simulink model "Track_model_wtihtesting_datacooling"  (R2024a)
settings: Solver=FixedStepAuto  StartTime=0.0  StopTime=1200  FixedStep=0.01  MaxStep=1e-2  MinStep=1e-5  RelTol=1e-3  AbsTol=1e-11
PreLoadFcn:
  | Straight1_Track = [75	3.446	29.063	1.834	47.653	8.247	3.373	13.154	57.193	39.54	5.916	3.204	2.701	2.747	90.673	4.72	3.366	94.658	23.788	1	40.161	15.969	17.891	3.717	36.358	76.419	54.208	36.993	4.775	55.007	1.783	4.349
  | ];
  | Curved_Track = [13.325	13.688	13.825	14.949	16.182	52.505	18.752	19.67	17.192	18.934	14.945	16.948	14.677	9.353	16.047	6.011	19.463	14.821	17.716	9.886	20.496	17.101	19.463	24.351	37.401	18.473	21.711	5.558	59.024	6.989	13.452	41.008
  | ];
  | Radius1 = [12	16.8	16.75	13.5	18.6	22.46	17.818	17.73	14	25.6	16.44	15.538	14.4	26.75	44.307	40	20.44	27.09	18.18	23.42	22.933	36.75	14.631	39	27.714	18.667	15.778	21.2	22.927	27.67	24.4	27.778
  | ];
model workspace (MAT data in the model file):
  Curve_Track = [19 13 16.3 21 23 16.5 21.6 28.81 24.6 43.9 54.836 13.8]
  Straight_Track = [35.7 53.5 32.527 50 30 20 11.2 36.6 21.4 41 38.7 74.5]
  Trac_vel = [10 5 8 12 8 9 10 9 11 14 10 10]
(part 1 of 2)
settings Model: Creator=91933  LastModifiedBy=Lenovo
settings SolverCC: MaxConsecutiveMinStep=10000000
settings DebuggingCC: UnconnectedInputMsg=warning  UnconnectedOutputMsg=warning  UnconnectedLineMsg=warning
settings ModelReferenceCC: EnableRefExpFcnMdlSchedulingChecks=on
settings RTWCC: GPUComputeCapability=3.5  DLArmComputeVersion=19.05

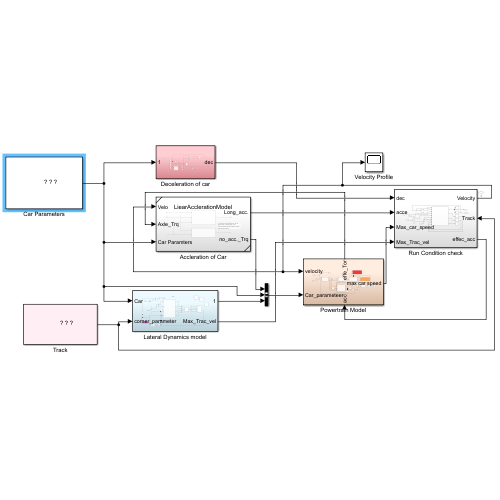
[thumbnail: Simulink's stored preview of the top-level diagram]
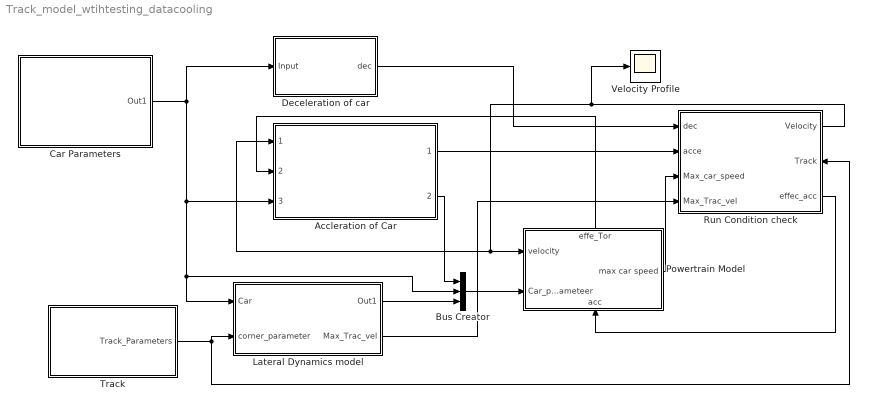
== system Track_model_wtihtesting_datacooling ==
  Accleration of Car : Subsystem  ReferencedSubsystem=LiearAcclerationModel
  Bus Creator : BusCreator  Inputs=3
  Car Parameters : Subsystem
      mask Display: image('C:\Users\91933\Pictures\IMG_5657.JPG'); % Use "Edit Image" on toolstrip to change.
  Deceleration of car : Subsystem
  Lateral Dynamics model : Subsystem
  Powertrain Model : Subsystem
      settings: PortSchema="{\"entries\":[{\"content\":{\"sides\":[{\"content\":{\"connectorIds\":[\"In1\",\"In2\"]},\"type\":\"ConnectorPlacement.EquallySpacedRectSide\",\"uuid\":\"7a6424a8-f57f-46b7-98ad-5f26a9320d27\"},{\"content\":{\"connectorIds\":[\"Out1\"],\"side\":\"RIGHT\"},\"type\":\"ConnectorPlacement.EquallySpacedRectSide\",\"uuid\":\"30370c1c-7325-4103-814a-5db3cbc3461c\"},{\"content\":{\"connectorIds\":[\"Out2\"],\"side\":\"TOP\"},\"type\":\"ConnectorPlacement.EquallySpacedRectSide\",\"uuid\":\"7e814e0a-36aa-401b-96b6-345dd2e08a66\"},{\"content\":{\"connectorIds\":[\"In3\"],\"side\":\"BOTTOM\"},\"type\":\"ConnectorPlacement.EquallySpacedRectSide\",\"uuid\":\"84f6999d-a613-4751-8b60-d9edc36e9be4\"}]},\"type\":\"ConnectorPlacement.EquallySpacedConnector\",\"uuid\":\"bd41e1c7-8fcc-402f-9d7e-0f9f747b7612\"}],\"packageUris\":[\"http://schema.mathworks.com/mf0/Connector/R2020b\"],\"version\":\"1.0\"}"
  Run Condition check : Subsystem
      settings: PortSchema="{\"entries\":[{\"content\":{\"sides\":[{\"content\":{\"connectorIds\":[\"In1\",\"In2\",\"In3\",\"In4\"]},\"type\":\"ConnectorPlacement.EquallySpacedRectSide\",\"uuid\":\"37420a10-33d8-4d00-9fe3-dd595a31418b\"},{\"content\":{\"connectorIds\":[\"Out1\",\"In5\",\"Out2\"],\"side\":\"RIGHT\"},\"type\":\"ConnectorPlacement.EquallySpacedRectSide\",\"uuid\":\"4603972b-d68c-4bfe-b153-0206992bf9a8\"},{\"content\":{\"connectorIds\":[],\"side\":\"TOP\"},\"type\":\"ConnectorPlacement.EquallySpacedRectSide\",\"uuid\":\"429b9389-e8bf-4c2b-b2c3-53413a2b6f78\"},{\"content\":{\"connectorIds\":[],\"side\":\"BOTTOM\"},\"type\":\"ConnectorPlacement.EquallySpacedRectSide\",\"uuid\":\"bf0772d6-0e04-49c3-b1e5-7cd72d464bde\"}]},\"type\":\"ConnectorPlacement.EquallySpacedConnector\",\"uuid\":\"b02c2900-baad-49e7-a583-da4e6719a609\"}],\"packageUris\":[\"http://schema.mathworks.com/mf0/Connector/R2020b\"],\"version\":\"1.0\"}"
  Track : Subsystem
      mask Display: image('Enduranc mdel.jpeg'); % Use "Edit Image" on toolstrip to change.
  Velocity Profile : Scope
  wires:
  Car Parameters/1(Out1) -> Deceleration of car/1(Input), Bus Creator/2, Lateral Dynamics model/1(Car), Accleration of Car/3
  Track/1(Track_Parameters) -> Run Condition check/5(Track), Lateral Dynamics model/2(corner_parameter)
  Lateral Dynamics model/2(Max_Trac_vel) -> Run Condition check/4(Max_Trac_vel)
  Powertrain Model/1(max car speed) -> Run Condition check/3(Max_car_speed)
  Bus Creator/1 -> Powertrain Model/2(Car_parameteer)
  Lateral Dynamics model/1(Out1) -> Bus Creator/3
  Deceleration of car/1(dec) -> Run Condition check/1(dec)
  Run Condition check/2(effec_acc) -> Powertrain Model/3(acc)
  Accleration of Car/2 -> Bus Creator/1
  Run Condition check/1(Velocity) -> Powertrain Model/1(velocity), Accleration of Car/1, Velocity Profile/1
  Accleration of Car/1 -> Run Condition check/2(acce)
  Powertrain Model/2(effe_Tor) -> Accleration of Car/2

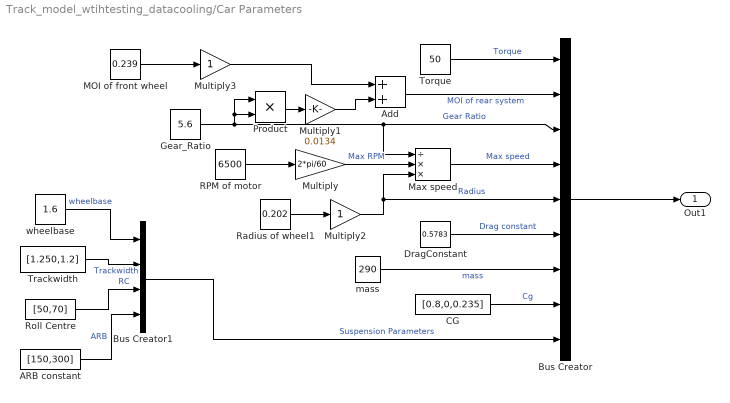
== system Track_model_wtihtesting_datacooling/Car Parameters ==
  ARB constant : Constant  Value=[150,300]
  Add : Sum
  Bus Creator : BusCreator  Inputs=9
  Bus Creator1 : BusCreator  Inputs=4
  "CG " : Constant  Value=[0.8,0,0.235]
  DragConstant : Constant  Value=0.5783
  Gear_Ratio : Constant  Value=5.6
  MOI of front wheel : Constant  Value=0.239
  Max speed : Product  Inputs=/**
  Multiply : Gain  Gain=2*pi/60
  Multiply1 : Gain  Gain=0.0134
  Multiply2 : Gain
  Multiply3 : Gain
  Product : Product
  RPM of motor : Constant  Value=6500
  Radius of wheel1 : Constant  Value=0.202
  Roll Centre : Constant  Value=[50,70]
  Torque : Constant  Value=50
  Trackwidth : Constant  Value=[1.250,1.2]
  mass : Constant  Value=290
  wheelbase : Constant  Value=1.6
  Out1 : Outport
  wires:
  Radius of wheel1/1 -> Multiply2/1
  mass/1 -> Bus Creator/7  "mass"
  Gear_Ratio/1 -> Max speed/1, Bus Creator/3, Product/2, Product/1  "Gear Ratio"
  Max speed/1 -> Bus Creator/4  "Max speed"
  DragConstant/1 -> Bus Creator/6  "Drag constant"
  Torque/1 -> Bus Creator/1  "Torque"
  Multiply/1 -> Max speed/2  "Max RPM"
  RPM of motor/1 -> Multiply/1
  Add/1 -> Bus Creator/2  "MOI of rear system"
  MOI of front wheel/1 -> Multiply3/1
  Product/1 -> Multiply1/1
  Multiply1/1 -> Add/2
  Multiply2/1 -> Max speed/3, Bus Creator/5  "Radius"
  Multiply3/1 -> Add/1
  "CG "/1 -> Bus Creator/8  "Cg"
  wheelbase/1 -> Bus Creator1/1  "wheelbase"
  Trackwidth/1 -> Bus Creator1/2  "Trackwidth"
  Roll Centre/1 -> Bus Creator1/3  "RC"
  ARB constant/1 -> Bus Creator1/4  "ARB"
  Bus Creator1/1 -> Bus Creator/9  "Suspension Parameters"
  Bus Creator/1 -> Out1/1

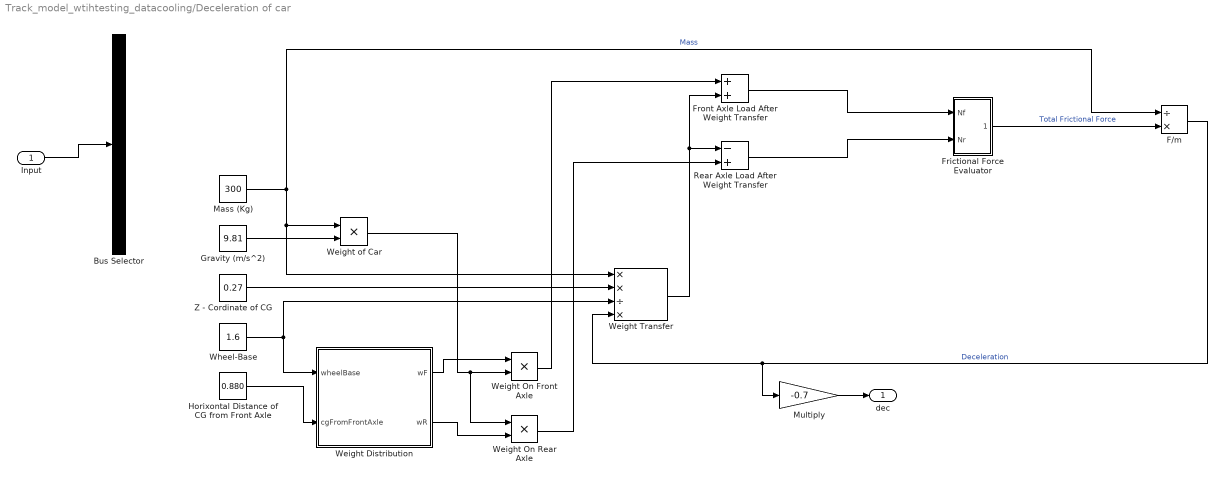
== system Track_model_wtihtesting_datacooling/Deceleration of car ==
  Input : Inport
  Bus Selector : BusSelector  OutputSignals=Torque,Gear Ratio,MOI of rear system,Radius,Drag constant,mass
  F/m : Product  Inputs=/*
  Frictional Force Evaluator : Subsystem
  Front Axle Load After Weight Transfer : Sum
  Gravity (m/s^2) : Constant  Value=9.81
  Horixontal Distance of CG from Front Axle : Constant  Value=0.880
  Mass (Kg) : Constant  Value=300
  Multiply : Gain  Gain=-0.7
  Rear Axle Load After Weight Transfer : Sum  Inputs=-+
  Weight Distribution : MATLAB Function  TreatAsAtomicUnit=on
  Weight On Front Axle : Product
  Weight On Rear Axle : Product
  Weight Transfer : Product  Inputs=**/*
  Weight of Car : Product
  Wheel-Base : Constant  Value=1.6
  Z - Cordinate of CG : Constant  Value=0.27
  dec : Outport
  wires:
  Input/1 -> Bus Selector/1
  Frictional Force Evaluator/1(Total F) -> F/m/2  "Total Frictional Force"
  Rear Axle Load After Weight Transfer/1 -> Frictional Force Evaluator/2(Nr)
  F/m/1 -> Multiply/1, Weight Transfer/4  "Deceleration"
  Wheel-Base/1 -> Weight Transfer/3, Weight Distribution/1(wheelBase)
  Front Axle Load After Weight Transfer/1 -> Frictional Force Evaluator/1(Nf)
  Z - Cordinate of CG/1 -> Weight Transfer/2
  Horixontal Distance of CG from Front Axle/1 -> Weight Distribution/2(cgFromFrontAxle)
  Weight On Rear Axle/1 -> Rear Axle Load After Weight Transfer/2
  Weight Transfer/1 -> Front Axle Load After Weight Transfer/2, Rear Axle Load After Weight Transfer/1
  Weight On Front Axle/1 -> Front Axle Load After Weight Transfer/1
  Mass (Kg)/1 -> Weight Transfer/1, Weight of Car/1, F/m/1  "Mass"
  Weight Distribution/1(wF) -> Weight On Front Axle/1
  Weight of Car/1 -> Weight On Rear Axle/1, Weight On Front Axle/2
  Weight Distribution/2(wR) -> Weight On Rear Axle/2
  Gravity (m/s^2)/1 -> Weight of Car/2
  Multiply/1 -> dec/1

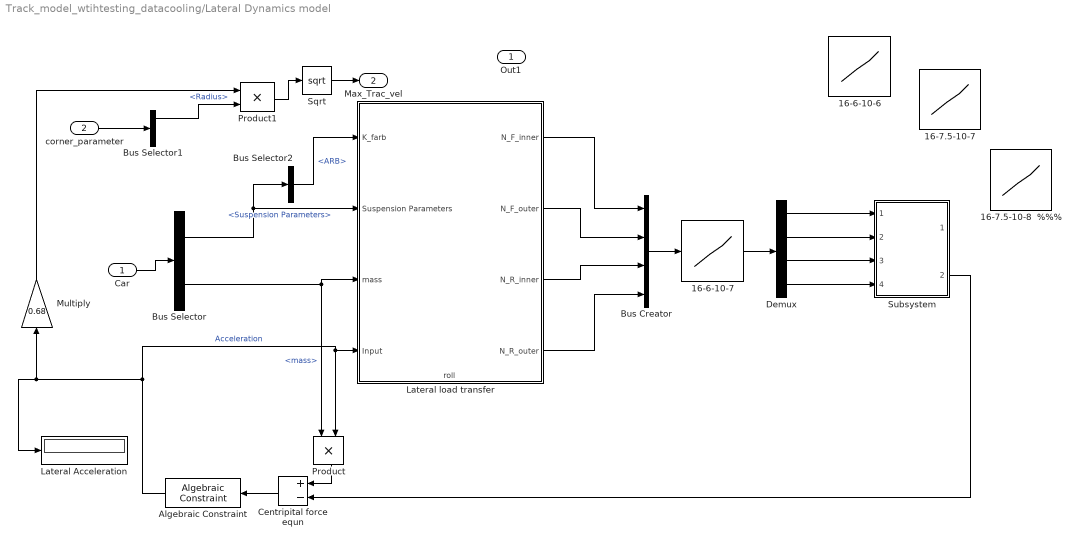
== system Track_model_wtihtesting_datacooling/Lateral Dynamics model ==
  Car : Inport
  corner_parameter : Inport  Port=2
  16-6-10-6 : Lookup_n-D  NumberOfTableDimensions=1  BreakpointsForDimension1="[300\t350\t400\t450\t500\t550\t600\t650\t700\t750\t800\t850\t900\t950\t1000\t1050\t1100\t1150\t1200\t1250]"  Table="[770\t888\t1000\t1114\t1223\t1329\t1437.73\t1536.3\t1633.67\t1731\t1825.46\t1911.31\t2002\t2086.06\t2166.12\t2247.6\t2320\t2385.38\t2457.68\t2520.95]"  InternalRulePriority=Speed  RndMeth=Simplest
  16-6-10-7 : Lookup_n-D  NumberOfTableDimensions=1  BreakpointsForDimension1="[210\t420\t660\t870\t1110]"  Table="[528.75\t1066\t1608\t2051\t2462.47]"  InternalRulePriority=Speed  RndMeth=Simplest
  16-7.5-10-7 : Lookup_n-D  NumberOfTableDimensions=1  BreakpointsForDimension1="[210\t420\t660\t870\t1110]"  Table="[660.96\t1204\t1721\t2247\t2672]"  InternalRulePriority=Speed  RndMeth=Simplest
  "16-7.5-10-8  %%% " : Lookup_n-D  NumberOfTableDimensions=1  BreakpointsForDimension1="[210\t420\t660\t870\t1110]"  Table="[557.43\t1141\t1671.36\t2190\t2663.17]"  InternalRulePriority=Speed  RndMeth=Simplest
  Algebraic Constraint : AlgebraicConstraint  InitialGuess=10
  Bus Creator : BusCreator  Inputs=4
  Bus Selector : BusSelector  OutputSignals=Suspension Parameters,mass
  Bus Selector1 : BusSelector  OutputSignals=Radius,CURVE
  Bus Selector2 : BusSelector  OutputSignals=ARB
  Centripital force equn : Sum  Inputs=+-
  Demux : Demux
  Lateral Acceleration : Display
  Lateral load transfer : Subsystem
      settings: PortSchema="{\"entries\":[{\"content\":{\"sides\":[{\"content\":{\"connectorIds\":[\"In1\",\"In2\",\"In3\",\"In4\"]},\"type\":\"ConnectorPlacement.EquallySpacedRectSide\",\"uuid\":\"21b7a285-463a-4549-b09f-31bf1463445a\"},{\"content\":{\"connectorIds\":[\"Out1\",\"Out2\",\"Out3\",\"Out4\"],\"side\":\"RIGHT\"},\"type\":\"ConnectorPlacement.EquallySpacedRectSide\",\"uuid\":\"9a065009-ffa8-4a15-bdfa-6b4336b1f24f\"},{\"content\":{\"connectorIds\":[],\"side\":\"TOP\"},\"type\":\"ConnectorPlacement.EquallySpacedRectSide\",\"uuid\":\"e0a28d16-0ef9-4a8b-b112-91cf0f57a153\"},{\"content\":{\"connectorIds\":[\"Out5\"],\"side\":\"BOTTOM\"},\"type\":\"ConnectorPlacement.EquallySpacedRectSide\",\"uuid\":\"92b5425f-e478-46c4-b62f-ee4f6d6d845d\"}]},\"type\":\"ConnectorPlacement.EquallySpacedConnector\",\"uuid\":\"77d231bd-30bb-4118-b341-ebc1a6567eef\"}],\"packageUris\":[\"http://schema.mathworks.com/mf0/Connector/R2020b\"],\"version\":\"1.0\"}"
  Multiply : Gain  Gain=0.68
  Product : Product
  Product1 : Product
  Sqrt : Sqrt
  Subsystem : Subsystem
  Out1 : Outport
  Max_Trac_vel : Outport  Port=2
  wires:
  corner_parameter/1 -> Bus Selector1/1
  Car/1 -> Bus Selector/1
  Centripital force equn/1 -> Algebraic Constraint/1
  Subsystem/2(Net force) -> Centripital force equn/2
  Product/1 -> Centripital force equn/1
  Bus Selector/1 -> Bus Selector2/1, Lateral load transfer/2(Suspension Parameters)  "<Suspension Parameters>"
  Bus Selector/2 -> Product/1, Lateral load transfer/3(mass)  "<mass>"
  Bus Selector2/1 -> Lateral load transfer/1(K_farb)  "<ARB>"
  Algebraic Constraint/1 -> Product/2, Lateral load transfer/4(Input), Lateral Acceleration/1, Multiply/1  "Acceleration"
  Bus Selector1/1 -> Product1/2  "<Radius>"
  Product1/1 -> Sqrt/1
  Sqrt/1 -> Max_Trac_vel/1
  Lateral load transfer/1(N_F_inner) -> Bus Creator/1
  Lateral load transfer/2(N_F_outer) -> Bus Creator/2
  Lateral load transfer/4(N_R_outer) -> Bus Creator/4
  Bus Creator/1 -> 16-6-10-7/1
  Lateral load transfer/3(N_R_inner) -> Bus Creator/3
  16-6-10-7/1 -> Demux/1
  Demux/1 -> Subsystem/1(N_F_inner)
  Demux/2 -> Subsystem/2(N_F_outer)
  Demux/3 -> Subsystem/3(N_R_inner)
  Demux/4 -> Subsystem/4(N_R_outer)
  Multiply/1 -> Product1/1

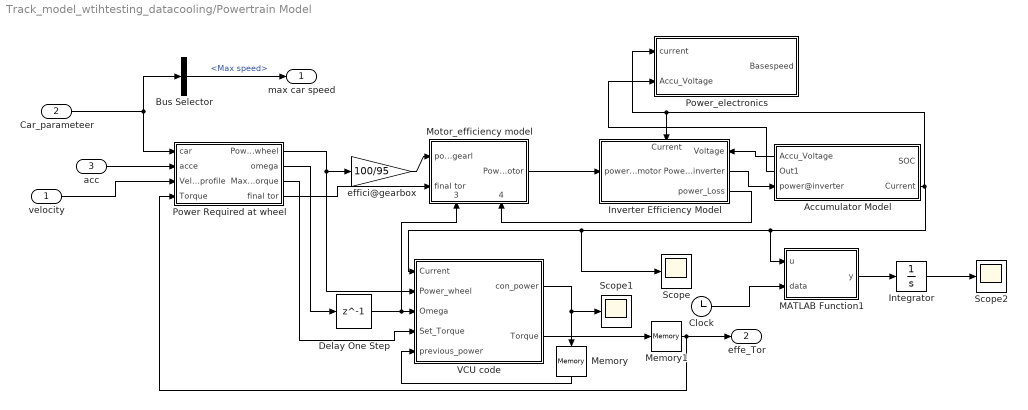
== system Track_model_wtihtesting_datacooling/Powertrain Model ==
  velocity : Inport
  Car_parameteer : Inport  Port=2
  acc : Inport  Port=3
  Accumulator Model : Subsystem
      settings: PortSchema="{\"entries\":[{\"content\":{\"sides\":[{\"content\":{\"connectorIds\":[\"Out3\",\"Out4\",\"In1\"]},\"type\":\"ConnectorPlacement.EquallySpacedRectSide\",\"uuid\":\"d9a2d271-dabe-4533-8ccb-f38955a31bcb\"},{\"content\":{\"connectorIds\":[\"Out1\",\"Out2\"],\"side\":\"RIGHT\"},\"type\":\"ConnectorPlacement.EquallySpacedRectSide\",\"uuid\":\"5b5f6e54-f39d-46a8-b35d-c03530deb970\"},{\"content\":{\"connectorIds\":[],\"side\":\"TOP\"},\"type\":\"ConnectorPlacement.EquallySpacedRectSide\",\"uuid\":\"8f799e0e-ee74-469a-8571-a72d5500dbda\"}]},\"type\":\"ConnectorPlacement.EquallySpacedConnector\",\"uuid\":\"33f1fb28-2aba-4ef3-a21b-2b6435cede70\"}],\"packageUris\":[\"http://schema.mathworks.com/mf0/Connector/R2020b\"],\"version\":\"1.0\"}"
  Bus Selector : BusSelector  OutputSignals=signal2.Max speed
  Clock : Clock
  Delay One Step : Delay  DelayLength=1
  Integrator : Integrator
  Inverter Efficiency Model : Subsystem
      settings: PortSchema="{\"entries\":[{\"content\":{\"sides\":[{\"content\":{\"connectorIds\":[\"In1\"]},\"type\":\"ConnectorPlacement.EquallySpacedRectSide\",\"uuid\":\"eeaf8c4c-ff4b-41f6-92ac-2ae23ce93843\"},{\"content\":{\"connectorIds\":[\"In3\",\"Out1\",\"Out2\"],\"side\":\"RIGHT\"},\"type\":\"ConnectorPlacement.EquallySpacedRectSide\",\"uuid\":\"c97de470-1590-4c04-99a9-b756f9e6d27c\"},{\"content\":{\"connectorIds\":[\"In2\"],\"side\":\"TOP\"},\"type\":\"ConnectorPlacement.EquallySpacedRectSide\",\"uuid\":\"61e260a0-3678-4462-9e97-077e8258dfd9\"}]},\"type\":\"ConnectorPlacement.EquallySpacedConnector\",\"uuid\":\"80720873-1fc3-4557-92cb-33646fe66d83\"}],\"packageUris\":[\"http://schema.mathworks.com/mf0/Connector/R2020b\"],\"version\":\"1.0\"}"
  MATLAB Function1 : MATLAB Function  TreatAsAtomicUnit=on
  Memory : Memory  InheritSampleTime=on  LinearizeMemory=on
  Memory1 : Memory  InitialCondition=50
  Motor_efficiency model : Subsystem
      settings: PortSchema="{\"entries\":[{\"content\":{\"sides\":[{\"content\":{\"connectorIds\":[\"In1\",\"In2\"]},\"type\":\"ConnectorPlacement.EquallySpacedRectSide\",\"uuid\":\"a939c6c9-94ea-465c-aed0-8455ff8139dc\"},{\"content\":{\"connectorIds\":[\"Out1\"],\"side\":\"RIGHT\"},\"type\":\"ConnectorPlacement.EquallySpacedRectSide\",\"uuid\":\"0f115e2b-b9ee-49f7-bcff-fb956452d489\"},{\"content\":{\"connectorIds\":[],\"side\":\"TOP\"},\"type\":\"ConnectorPlacement.EquallySpacedRectSide\",\"uuid\":\"fac63da4-7916-4207-9a64-f69c73a6da5b\"},{\"content\":{\"connectorIds\":[\"In3\",\"In4\"],\"side\":\"BOTTOM\"},\"type\":\"ConnectorPlacement.EquallySpacedRectSide\",\"uuid\":\"3a141222-bc99-40cd-96c4-ca0ab454ea99\"}]},\"type\":\"ConnectorPlacement.EquallySpacedConnector\",\"uuid\":\"67a82dfa-4075-49b0-ae40-d1da7dc236ad\"}],\"packageUris\":[\"http://schema.mathworks.com/mf0/Connector/R2020b\"],\"version\":\"1.0\"}"
  Power Required at wheel : Subsystem
  Power_electronics : Subsystem
  Scope : Scope
  Scope1 : Scope
  Scope2 : Scope
  VCU code : MATLAB Function  TreatAsAtomicUnit=on
  effici@gearbox : Gain  Gain=100/95
  max car speed : Outport
  effe_Tor : Outport  Port=2
  wires:
  Car_parameteer/1 -> Power Required at wheel/1(car), Bus Selector/1
  acc/1 -> Power Required at wheel/2(acce)
  velocity/1 -> Power Required at wheel/3(Velocity profile)
  Power Required at wheel/1(Power@wheel) -> VCU code/2(Power_wheel), effici@gearbox/1
  effici@gearbox/1 -> Motor_efficiency model/1(power@gearl)
  Inverter Efficiency Model/1(Power@inverter) -> Accumulator Model/1(power@inverter)
  Accumulator Model/2(Current) -> Power_electronics/1(current), Inverter Efficiency Model/2(Current), MATLAB Function1/1(u), Scope/1, VCU code/1(Current)
  Accumulator Model/3(Accu_Voltage) -> Inverter Efficiency Model/3(Voltage)
  Bus Selector/1 -> max car speed/1  "<Max speed>"
  VCU code/1(con_power) -> Scope1/1, Memory/1
  Memory/1 -> VCU code/5(previous_power)
  Power Required at wheel/3(Max_set torque) -> VCU code/4(Set_Torque)
  Power Required at wheel/2(omega) -> Delay One Step/1
  VCU code/2(Torque) -> Memory1/1
  Delay One Step/1 -> Motor_efficiency model/3(omega of wheel), VCU code/3(Omega)
  Memory1/1 -> Power Required at wheel/4(Torque), effe_Tor/1
  Accumulator Model/4(Out1) -> Power_electronics/2(Accu_Voltage)
  Motor_efficiency model/1(Power@motor) -> Inverter Efficiency Model/1(power@motor)
  Inverter Efficiency Model/2(power_Loss) -> Motor_efficiency model/4(inverter load)
  MATLAB Function1/1(y) -> Integrator/1
  Clock/1 -> MATLAB Function1/2(data)
  Integrator/1 -> Scope2/1
  Power Required at wheel/4(final tor) -> Motor_efficiency model/2(final tor)

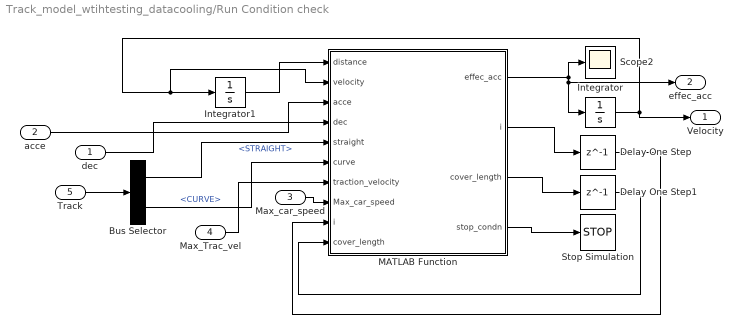
== system Track_model_wtihtesting_datacooling/Run Condition check ==
  dec : Inport
  acce : Inport  Port=2
  Max_car_speed : Inport  Port=3
  Max_Trac_vel : Inport  Port=4
  Track : Inport  Port=5
  Bus Selector : BusSelector  OutputSignals=STRAIGHT,CURVE
  Delay One Step : Delay  DelayLength=1
  Delay One Step1 : Delay  DelayLength=1
  Integrator : Integrator
  Integrator1 : Integrator
  MATLAB Function : MATLAB Function  TreatAsAtomicUnit=on
  Scope2 : Scope
  Stop Simulation : Stop
  Velocity : Outport
  effec_acc : Outport  Port=2
  wires:
  Integrator/1 -> MATLAB Function/2(velocity), Integrator1/1, Velocity/1
  MATLAB Function/2(i) -> Delay One Step/1
  MATLAB Function/1(effec_acc) -> Integrator/1, effec_acc/1, Scope2/1
  Integrator1/1 -> MATLAB Function/1(distance)
  Delay One Step1/1 -> MATLAB Function/10("cover_length ")
  Delay One Step/1 -> MATLAB Function/9("i ")
  MATLAB Function/4(stop_condn) -> Stop Simulation/1
  MATLAB Function/3(cover_length) -> Delay One Step1/1
  acce/1 -> MATLAB Function/3(acce)
  Track/1 -> Bus Selector/1
  Bus Selector/1 -> MATLAB Function/5(straight)  "<STRAIGHT>"
  Bus Selector/2 -> MATLAB Function/6(curve)  "<CURVE>"
  dec/1 -> MATLAB Function/4(dec)
  Max_Trac_vel/1 -> MATLAB Function/7(traction_velocity)
  Max_car_speed/1 -> MATLAB Function/8(Max_car_speed)

== system Track_model_wtihtesting_datacooling/Track ==
  Bus Creator : BusCreator  Inputs=3
  Constant : Constant  Value=Curved_Track
  Constant1 : Constant  Value=Straight1_Track
  Constant2 : Constant  Value=Radius1
  Track_Parameters : Outport
  wires:
  Constant/1 -> Bus Creator/2  "CURVE"
  Constant1/1 -> Bus Creator/1  "STRAIGHT"
  Constant2/1 -> Bus Creator/3  "Radius"
  Bus Creator/1 -> Track_Parameters/1

== system Track_model_wtihtesting_datacooling/Deceleration of car/Frictional Force Evaluator ==
  Nf : Inport
  Nr : Inport  Port=2
  F : Sum
  Friction Co-efficients : MATLAB Function  TreatAsAtomicUnit=on
  Front Axle : Gain  Gain=2
  Front Frictional Force Front Tyre : Product
  Multiply : Gain  Gain=0.5
  Multiply1 : Gain  Gain=0.5
  Rear Axle : Gain  Gain=2
  Rear Frictional Force Rear Tyre : Product
  Total F : Outport
  wires:
  Nr/1 -> Multiply1/1
  Rear Axle/1 -> F/2
  F/1 -> Total F/1
  Front Axle/1 -> F/1
  Front Frictional Force Front Tyre/1 -> Front Axle/1
  Multiply1/1 -> Rear Frictional Force Rear Tyre/2, Friction Co-efficients/2(Nr)
  Friction Co-efficients/2(uR) -> Rear Frictional Force Rear Tyre/1
  Friction Co-efficients/1(uF) -> Front Frictional Force Front Tyre/2
  Rear Frictional Force Rear Tyre/1 -> Rear Axle/1
  Multiply/1 -> Front Frictional Force Front Tyre/1, Friction Co-efficients/1(Nf)
  Nf/1 -> Multiply/1

== system Track_model_wtihtesting_datacooling/Lateral Dynamics model/Lateral load transfer ==
  K_farb : Inport
  Suspension Parameters : Inport  Port=2
  mass : Inport  Port=3
  Input : Inport  Port=4
  LATERAL LOAD TRANSFER : MATLAB Function  TreatAsAtomicUnit=on
  N_F_inner : Outport
  N_F_outer : Outport  Port=2
  N_R_inner : Outport  Port=3
  N_R_outer : Outport  Port=4
  roll : Outport  Port=5
  wires:
  LATERAL LOAD TRANSFER/1(N_F_inner) -> N_F_inner/1
  LATERAL LOAD TRANSFER/2(N_F_outer) -> N_F_outer/1
  K_farb/1 -> LATERAL LOAD TRANSFER/1(K_Arb)
  mass/1 -> LATERAL LOAD TRANSFER/2(mass)
  LATERAL LOAD TRANSFER/3(N_R_inner) -> N_R_inner/1
  LATERAL LOAD TRANSFER/4(N_R_outer) -> N_R_outer/1
  LATERAL LOAD TRANSFER/5(roll) -> roll/1
  Suspension Parameters/1 -> LATERAL LOAD TRANSFER/4(unused)
  Input/1 -> LATERAL LOAD TRANSFER/3(lateral_acc)

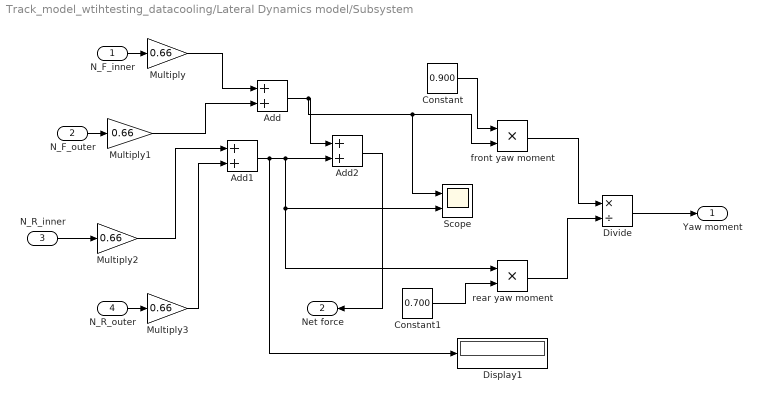
== system Track_model_wtihtesting_datacooling/Lateral Dynamics model/Subsystem ==
  N_F_inner : Inport
  N_F_outer : Inport  Port=2
  N_R_inner : Inport  Port=3
  N_R_outer : Inport  Port=4
  Add : Sum
  Add1 : Sum
  Add2 : Sum
  Constant : Constant  Value=0.900
  Constant1 : Constant  Value=0.700
  Display1 : Display
  Divide : Product  Inputs=*/
  Multiply{,1..3} (4 alike) : Gain  Gain=0.66
  Scope : Scope  NumInputPorts=2
  front yaw moment : Product
  rear yaw moment : Product
  "Yaw moment " : Outport
  Net force : Outport  Port=2
  wires:
  N_R_inner/1 -> Multiply2/1
  N_F_outer/1 -> Multiply1/1
  N_F_inner/1 -> Multiply/1
  Add2/1 -> Net force/1
  N_R_outer/1 -> Multiply3/1
  Constant1/1 -> rear yaw moment/2
  Add1/1 -> Display1/1, Scope/2, rear yaw moment/1, Add2/2
  Add/1 -> Scope/1, front yaw moment/2, Add2/1
  Constant/1 -> front yaw moment/1
  front yaw moment/1 -> Divide/1
  rear yaw moment/1 -> Divide/2
  Divide/1 -> "Yaw moment "/1
  Multiply/1 -> Add/1
  Multiply3/1 -> Add1/2
  Multiply2/1 -> Add1/1
  Multiply1/1 -> Add/2

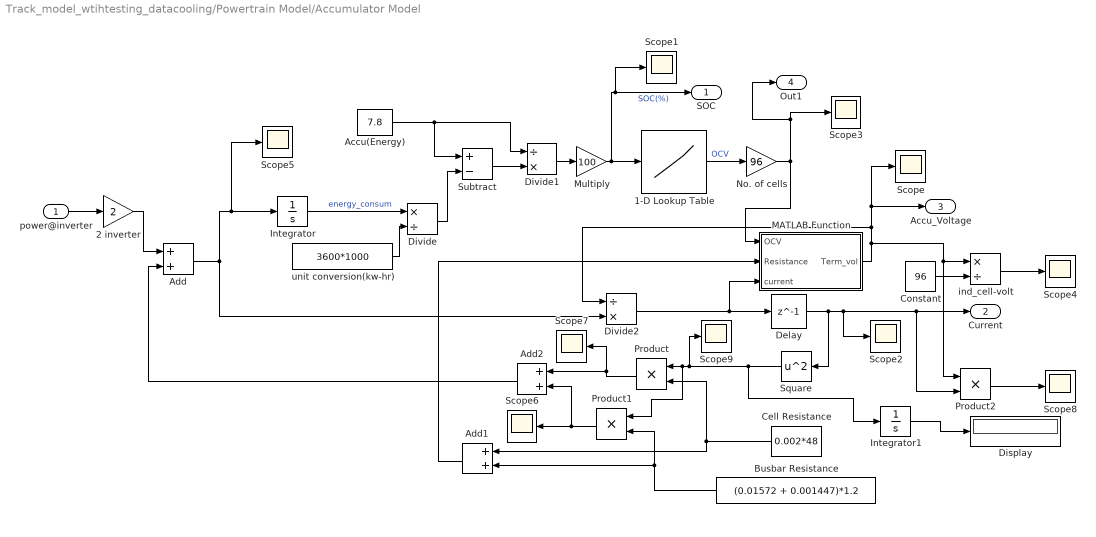
== system Track_model_wtihtesting_datacooling/Powertrain Model/Accumulator Model ==
  power@inverter : Inport
  1-D Lookup Table : Lookup_n-D  NumberOfTableDimensions=1  BreakpointsForDimension1="[6.39\t7\t8\t9\t10\t11\t12\t13\t14\t15\t16\t17\t18\t19\t20\t21\t22\t23\t24\t25\t26\t27\t28\t29\t30\t31\t32\t33\t34\t35\t36\t37\t38\t39\t40\t41\t42\t43\t44\t45\t46\t47\t48\t49\t50\t51\t52\t53\t54\t55\t56\t57\t58\t59\t60\t61\t62\t63\t64\t65\t66\t67\t68\t69\t70\t71\t72\t73\t74\t75\t76\t77\t78\t79\t80\t81\t82\t83\t84\t85\t86\t87\t88\t89\t90\t91\t92\t93\t94\t95\t96\t97\t98\t99\t100]"  Table="[3\t3.2415\t3.3884\t3.4785\t3.5428\t3.5919\t3.6311\t3.6585\t3.6678\t3.6719\t3.6741\t3.6759\t3.6774\t3.6791\t3.6838\t3.692\t3.6984\t3.7031\t3.7072\t3.7118\t3.717\t3.7211\t3.7249\t3.7282\t3.7312\t3.7339\t3.7372\t3.7406\t3.744\t3.7478\t3.7504\t3.7529\t3.7553\t3.7577\t3.7595\t3.761\t3.7629\t3.7647\t3.7668\t3.7684\t3.7707\t3.7726\t3.7748\t3.7772\t3.7795\t3.7819\t3.7844\t3.7871\t3.7896\t3.7931\t3.7962\t3.7995\t3.8031\t3.8073\t3.8114\t3.8158\t3.8206\t3.8253\t3.8304\t3.8358\t3.8411\t3.8473\t3.8541\t3.8616\t3.8699\t3.8785\t3.8865\t3.8939\t3.9011\t3.9075\t3.9137\t3.92\t3.9261\t3.9327\t3.9396\t3.9457\t3.9509\t3.9554\t3.9597\t3.9642\t3.9701\t3.9777\t3.9857\t3.9959\t4.0086\t4.025\t4.0422\t4.0549\t4.0629\t4.068\t4.0727\t4.0798\t4.0873\t4.0969\t4.116]"  InternalRulePriority=Speed  RndMeth=Simplest
  2 inverter : Gain  Gain=2
  Accu(Energy) : Constant  Value=7.8
  Add : Sum
  Add1 : Sum
  Add2 : Sum
  Busbar Resistance : Constant  Value=(0.01572 + 0.001447)*1.2
  Cell Resistance : Constant  Value=0.002*48
  Constant : Constant  Value=96
  Delay : Delay  DelayLength=1
  Display : Display
  Divide : Product  Inputs=*/
  Divide1 : Product  Inputs=/*
  Divide2 : Product  Inputs=/*
  Integrator : Integrator
  Integrator1 : Integrator
  MATLAB Function : MATLAB Function  TreatAsAtomicUnit=on
  Multiply : Gain  Gain=100
  No. of cells : Gain  Gain=96
  Product : Product
  Product1 : Product
  Product2 : Product
  Scope{,1..9} (10 alike) : Scope
  Square : Math  Operator=square
  Subtract : Sum  Inputs=+-
  ind_cell-volt : Product  Inputs=*/
  unit conversion(kw-hr) : Constant  Value=3600*1000
  SOC : Outport
  Current : Outport  Port=2
  Accu_Voltage : Outport  Port=3
  Out1 : Outport  Port=4
  wires:
  power@inverter/1 -> 2 inverter/1
  Accu(Energy)/1 -> Divide1/1, Subtract/1
  Integrator/1 -> Divide/1  "energy_consum"
  unit conversion(kw-hr)/1 -> Divide/2
  Divide/1 -> Subtract/2
  Subtract/1 -> Divide1/2
  1-D Lookup Table/1 -> No. of cells/1  "OCV"
  Divide1/1 -> Multiply/1
  Multiply/1 -> Scope1/1, SOC/1, 1-D Lookup Table/1  "SOC(%)"
  Divide2/1 -> Delay/1, MATLAB Function/3(current)
  No. of cells/1 -> Out1/1, Scope3/1, MATLAB Function/1(OCV)
  2 inverter/1 -> Add/1
  MATLAB Function/1(Term_vol) -> Product2/1, ind_cell-volt/1, Scope/1, Accu_Voltage/1, Divide2/1
  Delay/1 -> Square/1, Scope2/1, Product2/2, Current/1
  Square/1 -> Integrator1/1, Scope9/1, Product1/1, Product/1
  Add2/1 -> Add/2
  Add/1 -> Divide2/2, Scope5/1, Integrator/1
  Constant/1 -> ind_cell-volt/2
  ind_cell-volt/1 -> Scope4/1
  Cell Resistance/1 -> Product/2, Add1/1
  Busbar Resistance/1 -> Product1/2, Add1/2
  Add1/1 -> MATLAB Function/2(Resistance)
  Product/1 -> Scope7/1, Add2/1
  Product1/1 -> Scope6/1, Add2/2
  Product2/1 -> Scope8/1
  Integrator1/1 -> Display/1

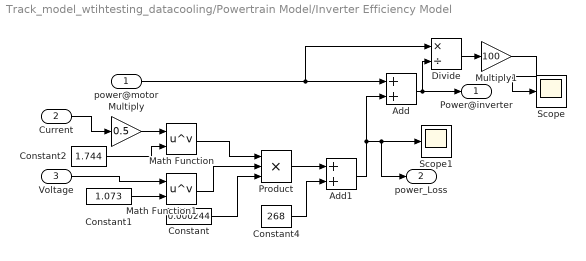
== system Track_model_wtihtesting_datacooling/Powertrain Model/Inverter Efficiency Model ==
  power@motor : Inport
  Current : Inport  Port=2
  Voltage : Inport  Port=3
  Add : Sum
  Add1 : Sum
  Constant : Constant  Value=0.000244
  Constant1 : Constant  Value=1.073
  Constant2 : Constant  Value=1.744
  Constant4 : Constant  Value=268
  Divide : Product  Inputs=*/
  Math Function : Math  Operator=pow
  Math Function1 : Math  Operator=pow
  Multiply : Gain  Gain=0.5
  Multiply1 : Gain  Gain=100
  Product : Product  Inputs=3
  Scope : Scope
  Scope1 : Scope
  Power@inverter : Outport
  power_Loss : Outport  Port=2
  wires:
  power@motor/1 -> Divide/1, Add/1
  Current/1 -> Multiply/1
  Constant2/1 -> Math Function/2
  Voltage/1 -> Math Function1/1
  Constant1/1 -> Math Function1/2
  Math Function/1 -> Product/1
  Math Function1/1 -> Product/2
  Constant/1 -> Product/3
  Product/1 -> Add1/1
  Constant4/1 -> Add1/2
  Add1/1 -> power_Loss/1, Scope1/1, Add/2
  Add/1 -> Divide/2, Power@inverter/1
  Multiply/1 -> Math Function/1
  Divide/1 -> Multiply1/1
  Multiply1/1 -> Scope/1

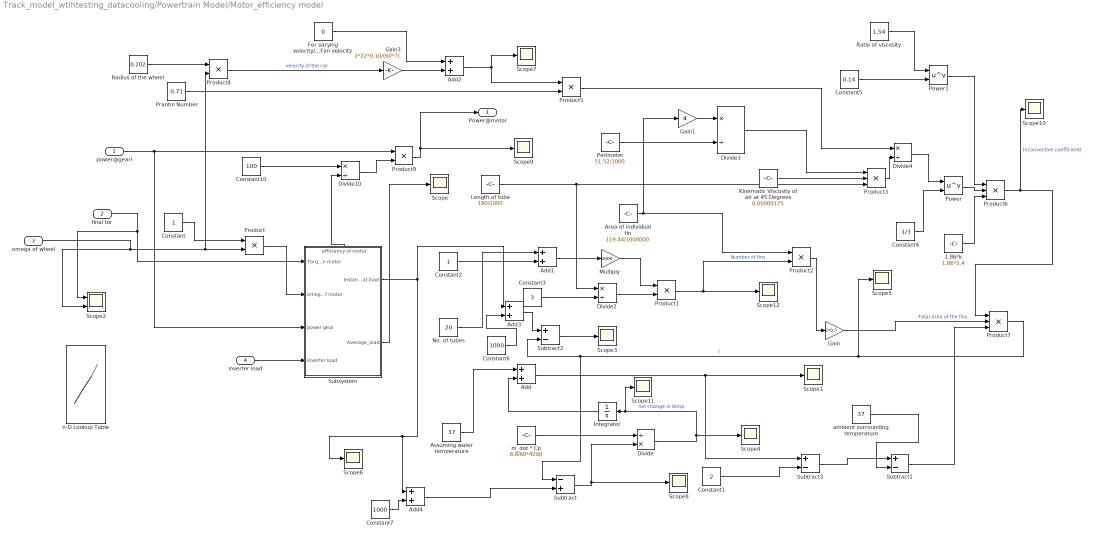
== system Track_model_wtihtesting_datacooling/Powertrain Model/Motor_efficiency model ==
  power@gearl : Inport
  final tor : Inport  Port=2
  omega of wheel : Inport  Port=3
  inverter load : Inport  Port=4
  1.86*k : Constant  Value=1.86*1.4
  Add{,1..4} (5 alike) : Sum
  Area of individual fin : Constant  Value=119.44/1000000
  Assuming water temperature : Constant  Value=37
  Constant : Constant
  Constant1 : Constant  Value=2
  Constant10 : Constant  Value=100
  Constant2 : Constant
  Constant3 : Constant  Value=3
  Constant4 : Constant  Value=1/3
  Constant5 : Constant  Value=0.14
  Constant6 : Constant  Value=1000
  Constant7 : Constant  Value=1000
  Divide : Product  Inputs=/*
  Divide{2..4,10} (4 alike) : Product  Inputs=*/
  For varying velocity/Fan velocity : Constant  Value=0
  Gain : Gain  Gain=2*0.5
  Gain1 : Gain  Gain=4
  Gain3 : Gain  Gain=2*22*0.10/(60*7)
  Integrator : Integrator
  Kinematic Viscosity of air at 45 Degrees : Constant  Value=0.00000175
  Length of tube : Constant  Value=180/1000
  Multiply : Gain  Gain=2000
  No. of tubes : Constant  Value=20
  Perimeter : Constant  Value=51.52/1000
  Power : Math  Operator=pow
  Power1 : Math  Operator=pow
  Prantnl Number : Constant  Value=0.71
  Product{,1..2,4..5,9} (6 alike) : Product
  Product3 : Product  Inputs=3
  Product6 : Product  Inputs=3
  Product7 : Product  Inputs=3
  Radius of the wheel : Constant  Value=0.202
  Ratio of viscosity : Constant  Value=1.54
  Scope{,1,3..12} (12 alike) : Scope
  Scope2 : Scope  NumInputPorts=2
  Subsystem : Subsystem
      settings: PortSchema="{\"entries\":[{\"content\":{\"sides\":[{\"content\":{\"connectorIds\":[\"In1\",\"In2\",\"In3\",\"In4\"]},\"type\":\"ConnectorPlacement.EquallySpacedRectSide\",\"uuid\":\"2b852e23-bbc1-45dd-844a-0e37338e81c6\"},{\"content\":{\"connectorIds\":[\"Out1\",\"Out2\"],\"side\":\"RIGHT\"},\"type\":\"ConnectorPlacement.EquallySpacedRectSide\",\"uuid\":\"37c03911-d7ce-4d3a-8358-a07da015470d\"},{\"content\":{\"connectorIds\":[\"Out3\"],\"side\":\"TOP\"},\"type\":\"ConnectorPlacement.EquallySpacedRectSide\",\"uuid\":\"eee8b6bb-27e3-4579-a0d8-2a4321e0e1a1\"}]},\"type\":\"ConnectorPlacement.EquallySpacedConnector\",\"uuid\":\"3ac61202-71cb-4132-bc22-f01fa752e354\"}],\"packageUris\":[\"http://schema.mathworks.com/mf0/Connector/R2020b\"],\"version\":\"1.0\"}"
  Subtract : Sum  Inputs=-+
  Subtract1 : Sum  Inputs=+-
  Subtract2 : Sum  Inputs=+-
  Subtract3 : Sum  Inputs=+-
  "ambient surrounding temperature " : Constant  Value=37
  m_dot * Cp : Constant  Value=8.8/60*4200
  n-D Lookup Table : Lookup_n-D  NumberOfTableDimensions=3  BreakpointsForDimension1=[150;190]  BreakpointsForDimension2=[20;28]  BreakpointsForDimension3=[30 31 32 33 34 35 36 37 38 39 40 41 42 43 44 45 46 47]  Table=reshape([0 0 0 0 67.25 83 88.25161 104 135 174 161 200 184.5 259 257 331.5 236.17 339 320.5 423.33 297.36 410 390.16 502.8 363.3 490 470.3 597 435 558 534 657 450.5 606.5 584 740.33 461.34 657.5 637.5 833.66 566.5 713 729.5 876 576.2 743 794 960.8 532.5 762 848.5 1078 534.15 815.9 881.5 1163.25 591.1 873.6 921.5 1204 637.4 920.9 977.5 1261 675.3 963.8 1033.5 1322 791.6 1006.6 1157 1372], [2 2 18])  InternalRulePriority=Speed  RndMeth=Simplest
      settings: InputPortMap=u0,u1,u2
  Power@motor : Outport
  wires:
  Product9/1 -> Power@motor/1, Scope9/1
  power@gearl/1 -> Subsystem/3(power gear), Product9/1
  Constant10/1 -> Divide10/1
  Subsystem/3(efficiency of motor) -> Divide10/2
  Divide10/1 -> Product9/2
  inverter load/1 -> Subsystem/4(inverter load)
  Subsystem/1(Instant Heat load) -> Add3/1, Add4/1, Scope6/1
  Subsystem/2(Average_load) -> Scope/1
  final tor/1 -> Scope2/1, Subsystem/1(Torque in motor)
  Length of tube/1 -> Divide2/1, Product3/3
  No. of tubes/1 -> Add1/1
  Subtract/1 -> Scope8/1, Divide/2
  m_dot * Cp/1 -> Divide/1
  omega of wheel/1 -> Scope2/2, Product4/2, Product/2
  Constant/1 -> Product/1
  Product/1 -> Subsystem/2(omegaof motor)
  Assuming water temperature/1 -> Add/1
  Constant3/1 -> Divide2/2
  Divide2/1 -> Product1/2
  Multiply/1 -> Product1/1
  Product1/1 -> Scope12/1, Product2/2  "Number of fins"
  Area of individual fin/1 -> Product2/1, Gain1/1
  Product2/1 -> Gain/1
  Gain1/1 -> Divide3/1
  Perimeter/1 -> Divide3/2
  Divide3/1 -> Product3/1
  Kinematic Viscosity of air at 45 Degrees/1 -> Product3/2
  Radius of the wheel/1 -> Product4/1
  Product4/1 -> Gain3/1  "velocity of the car"
  Prantnl Number/1 -> Product5/2
  Product5/1 -> Divide4/1
  Product3/1 -> Divide4/2
  Divide4/1 -> Power/1
  Constant4/1 -> Power/2
  Ratio of viscosity/1 -> Power1/1
  Constant5/1 -> Power1/2
  Power1/1 -> Product6/1
  Power/1 -> Product6/2
  1.86*k/1 -> Product6/3
  Gain/1 -> Product7/2  "Total Area of the fins"
  Product6/1 -> Scope10/1, Product7/1  "h(convective coefficient)"
  Product7/1 -> Subtract/1, Subtract2/2, Scope5/1  "l"
  Subtract2/1 -> Scope3/1
  Constant2/1 -> Add1/2
  Add1/1 -> Multiply/1
  For varying velocity/Fan velocity/1 -> Add2/1
  Add2/1 -> Product5/1, Scope7/1
  Gain3/1 -> Add2/2
  Divide/1 -> Scope11/1, Integrator/1, Scope4/1  "net change in temp"
  Subtract1/1 -> Product7/3
  Add/1 -> Scope1/1, Subtract3/1
  Integrator/1 -> Add/2
  "ambient surrounding temperature "/1 -> Subtract1/2
  Constant1/1 -> Subtract3/2
  Subtract3/1 -> Subtract1/1
  Constant6/1 -> Add3/2
  Add3/1 -> Subtract2/1
  Constant7/1 -> Add4/2
  Add4/1 -> Subtract/2

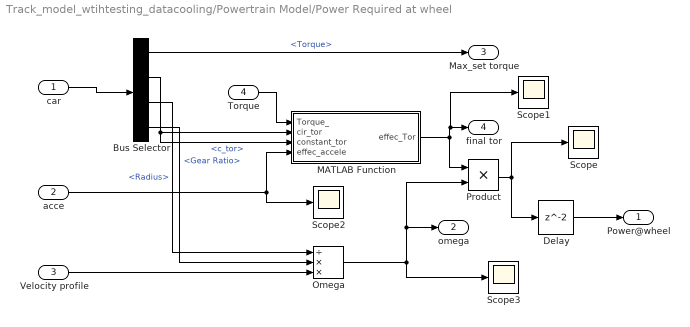
== system Track_model_wtihtesting_datacooling/Powertrain Model/Power Required at wheel ==
  car : Inport
  acce : Inport  Port=2
  Velocity profile : Inport  Port=3
  Torque : Inport  Port=4
  Bus Selector : BusSelector  OutputSignals=signal2.Torque,c_tor,signal2.Radius,signal2.Gear Ratio
  Delay : Delay
  MATLAB Function : MATLAB Function  TreatAsAtomicUnit=on
  Omega : Product  Inputs=/**
  Product : Product
  Scope{,1..3} (4 alike) : Scope
  Power@wheel : Outport
  omega : Outport  Port=2
  Max_set torque : Outport  Port=3
  final tor : Outport  Port=4
  wires:
  Bus Selector/1 -> Max_set torque/1  "<Torque>"
  Bus Selector/2 -> MATLAB Function/3(constant_tor), MATLAB Function/2(cir_tor)  "<c_tor>"
  Bus Selector/3 -> Omega/1  "<Radius>"
  Omega/1 -> omega/1, Product/2, Scope3/1
  Bus Selector/4 -> Omega/2  "<Gear Ratio>"
  MATLAB Function/1(effec_Tor) -> Product/1, Scope1/1, final tor/1
  acce/1 -> MATLAB Function/4(effec_accele), Scope2/1
  car/1 -> Bus Selector/1
  Velocity profile/1 -> Omega/3
  Torque/1 -> MATLAB Function/1(Torque_)
  Product/1 -> Delay/1, Scope/1
  Delay/1 -> Power@wheel/1

== system Track_model_wtihtesting_datacooling/Powertrain Model/Power_electronics ==
  current : Inport
  Accu_Voltage : Inport  Port=2
  MATLAB Function : MATLAB Function  TreatAsAtomicUnit=on
  Scope : Scope  NumInputPorts=2
  Basespeed : Outport
  wires:
  current/1 -> MATLAB Function/2(Idc)
  MATLAB Function/1(Base_speed) -> Scope/1, Basespeed/1
  Accu_Voltage/1 -> MATLAB Function/1(Vdc)
